simulink model "zbt_transpose"  (Simulink 6.2)
settings: Solver=ode45  StartTime=0.0  StopTime=10.0  RelTol=1e-3
libraries: xbsIndex_r3 x90, fb_library x4
settings Model: LastModifiedBy=mdexter
settings DebuggingCC: SolverPrmCheckMsg=warning

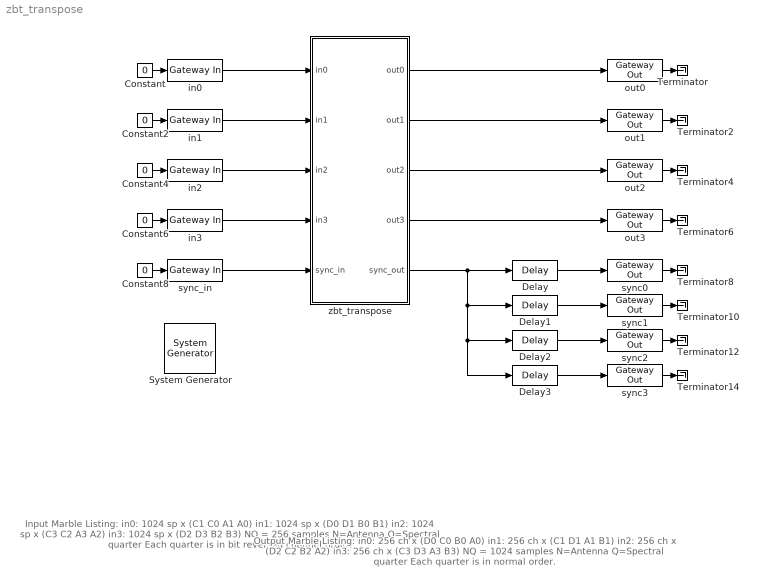
== system zbt_transpose ==
  note: Input Marble Listing:
      |
      | in0: 1024 sp x (C1 C0 A1 A0)
      | in1: 1024 sp x (D0 D1 B0 B1)
      | in2: 1024 sp x (C3 C2 A3 A2)
      | in3: 1024 sp x (D2 D3 B2 B3)
      |
      | NQ = 256 samples
      |
      | N=Antenna
      | Q=Spectral quarter
      |
      | Each quarter is in bit
      | reversed channel order.
  note: Output Marble Listing:
      |
      | in0: 256 ch x (D0 C0 B0 A0)
      | in1: 256 ch x (C1 D1 A1 B1)
      | in2: 256 ch x (D2 C2 B2 A2)
      | in3: 256 ch x (C3 D3 A3 B3)
      |
      | NQ = 1024 samples
      |
      | N=Antenna
      | Q=Spectral quarter
      |
      | Each quarter is in
      | normal order.
  " System Generator" : xbsIndex_r3/ System Generator  Tag=genX  xilinxfamily=Virtex2P  part=xc2vp40  speed=-6  package=ff1152  synthesis_tool=XST  directory=./zbt_transpose_core  testbench=off  simulink_period=1  sysclk_period=100  incr_netlist=off  trim_vbits=Everywhere in SubSystem  dbl_ovrd=According to Block Masks  core_generation=According to Block Masks  run_coregen=off  deprecated_control=off  eval_field=0
      settings: AttributesFormatString=System\nGenerator
  Constant{,2,4,6,8} (5 alike) : Constant  Value=0
  Delay{,1..3} (4 alike) : xbsIndex_r3/Delay  latency=1  reg_retiming=off  explicit_period=off  period=1  en=off  accept_only_valid=off  init_zero=on  dbl_ovrd=off  show_param=off
      settings: xl_area=[0, 0, 0, 0, 0, 0, 0]
  Terminator{,2,4,6,8,10,12,14} (8 alike) : Terminator
  in{0..3} (4 alike) : xbsIndex_r3/Gateway In  arith_type=Unsigned  n_bits=16  bin_pt=0  quantization=Truncate  overflow=Wrap  period=1  timing_constraint=None  locs_specified=off  LOCs={}  needs_fixed_name=off  dbl_ovrd=off  show_param=off
      settings: xl_area=[0, 0, 0, 0, 0, 0, 0]
  out{0..3} (4 alike) : xbsIndex_r3/Gateway Out  output_type=Double  nbits=8  bin_pt=6  arith_type=Boolean  quantization=Truncate  overflow=Wrap  hdl_port=on  timing_constraint=None  locs_specified=off  LOCs={}  needs_fixed_name=off  show_param=off
      settings: xl_area=[0, 0, 0, 0, 0, 0, 0]
  sync{0..3} (4 alike) : xbsIndex_r3/Gateway Out  output_type=Double  nbits=8  bin_pt=6  arith_type=Boolean  quantization=Truncate  overflow=Wrap  hdl_port=on  timing_constraint=None  locs_specified=off  LOCs={}  needs_fixed_name=off  show_param=off
      settings: xl_area=[0, 0, 0, 0, 0, 0, 0]
  sync_in : xbsIndex_r3/Gateway In  arith_type=Boolean  n_bits=16  bin_pt=0  quantization=Truncate  overflow=Wrap  period=1  timing_constraint=None  locs_specified=off  LOCs={}  needs_fixed_name=off  dbl_ovrd=off  show_param=off
      settings: xl_area=[0, 0, 0, 0, 0, 0, 0]
  zbt_transpose : Subsystem
  wires:
  sync_in/1 -> zbt_transpose/5(sync_in)
  zbt_transpose/5(sync_out) -> Delay/1, Delay1/1, Delay3/1, Delay2/1
  Delay/1 -> sync0/1
  Delay1/1 -> sync1/1
  Delay2/1 -> sync2/1
  Delay3/1 -> sync3/1
  Constant/1 -> in0/1
  Constant2/1 -> in1/1
  Constant4/1 -> in2/1
  Constant6/1 -> in3/1
  Constant8/1 -> sync_in/1
  out0/1 -> Terminator/1
  out1/1 -> Terminator2/1
  out2/1 -> Terminator4/1
  out3/1 -> Terminator6/1
  sync0/1 -> Terminator8/1
  sync1/1 -> Terminator10/1
  sync2/1 -> Terminator12/1
  sync3/1 -> Terminator14/1
  in0/1 -> zbt_transpose/1(in0)
  in1/1 -> zbt_transpose/2(in1)
  in2/1 -> zbt_transpose/3(in2)
  in3/1 -> zbt_transpose/4(in3)
  zbt_transpose/1(out0) -> out0/1
  zbt_transpose/2(out1) -> out1/1
  zbt_transpose/3(out2) -> out2/1
  zbt_transpose/4(out3) -> out3/1

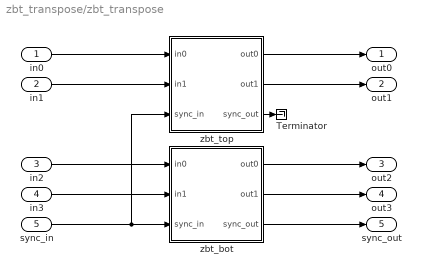
== system zbt_transpose/zbt_transpose ==
  in0 : Inport  Port=1  LatchInput=off
  in1 : Inport  Port=2  LatchInput=off
  in2 : Inport  Port=3  LatchInput=off
  in3 : Inport  Port=4  LatchInput=off
  sync_in : Inport  Port=5  LatchInput=off
  Terminator : Terminator
  zbt_bot : Subsystem
  zbt_top : Subsystem
  out0 : Outport
  out1 : Outport  Port=2
  out2 : Outport  Port=3
  out3 : Outport  Port=4
  sync_out : Outport  Port=5
  wires:
  zbt_top/1(out0) -> out0/1
  in0/1 -> zbt_top/1(in0)
  in1/1 -> zbt_top/2(in1)
  zbt_top/2(out1) -> out1/1
  zbt_bot/1(out0) -> out2/1
  in2/1 -> zbt_bot/1(in0)
  in3/1 -> zbt_bot/2(in1)
  zbt_bot/2(out1) -> out3/1
  sync_in/1 -> zbt_bot/3(sync_in), zbt_top/3(sync_in)
  zbt_bot/3(sync_out) -> sync_out/1
  zbt_top/3(sync_out) -> Terminator/1

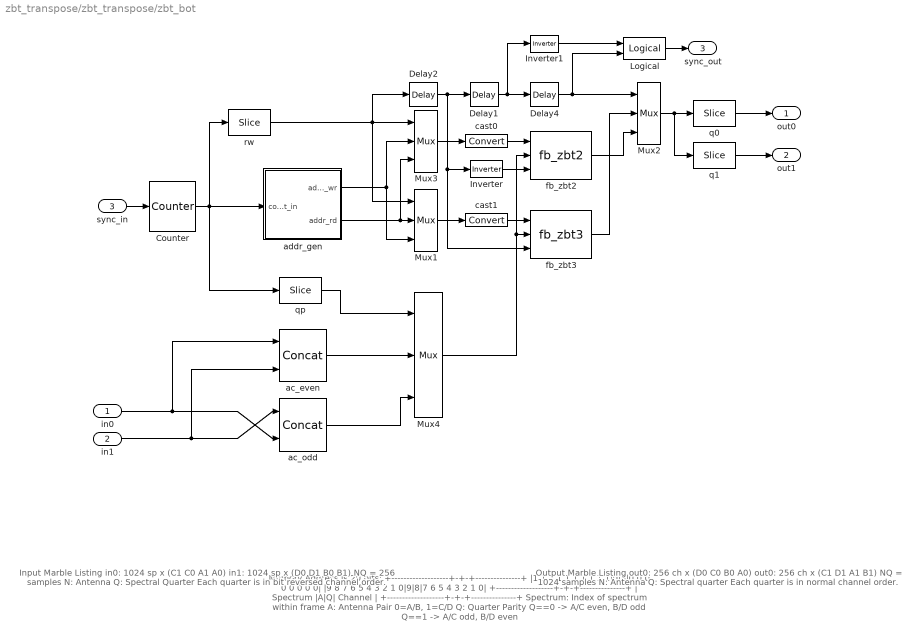
== system zbt_transpose/zbt_transpose/zbt_bot ==
  note: Memory Address is 20 bits:
      | +-------------------+-+-+---------------+
      | |1 1 1 1 1 1 1 1 1 1|0|0|0 0 0 0 0 0 0 0|
      | |9 8 7 6 5 4 3 2 1 0|9|8|7 6 5 4 3 2 1 0|
      | +-------------------+-+-+---------------+
      | |     Spectrum      |A|Q|    Channel    |
      | +-------------------+-+-+---------------+
      |
      | Spectrum: Index of spectrum within frame
      | A: Antenna Pair 0=A/B, 1=C/D
      | Q: Quarter Parity
      | Q==0 -> A/C even, B/D odd
      | Q==1 -> A/C odd, B/D even
  note: Input Marble Listing
      | in0: 1024 sp x (C1 C0 A1 A0)
      | in1: 1024 sp x (D0 D1 B0 B1)
      |
      | NQ = 256 samples
      |
      | N: Antenna
      | Q: Spectral Quarter
      |
      | Each quarter is in bit
      | reversed channel order.
  note: Output Marble Listing
      | out0: 256 ch x (D0 C0 B0 A0)
      | out0: 256 ch x (C1 D1 A1 B1)
      |
      | NQ = 1024 samples
      |
      | N: Antenna
      | Q: Spectral quarter
      |
      | Each quarter is in
      | normal channel order.
  in0 : Inport  Port=1  LatchInput=off
  in1 : Inport  Port=2  LatchInput=off
  sync_in : Inport  Port=3  LatchInput=off
  Counter : xbsIndex_r3/Counter  cnt_type=Free Running  n_bits=21  bin_pt=0  arith_type=Unsigned  start_count=0  cnt_to=Inf  cnt_by_val=1  operation=Up  explicit_period=on  period=1  load_pin=off  rst=on  en=off  dbl_ovrd=off  show_param=off  use_rpm=on  gen_core=off
      settings: xl_area=[0, 0, 0, 0, 0, 0, 0]
  Delay1 : xbsIndex_r3/Delay  latency=3  reg_retiming=off  explicit_period=off  period=1  en=off  accept_only_valid=off  init_zero=on  dbl_ovrd=off  show_param=off
      settings: xl_area=[0, 0, 0, 0, 0, 0, 0]
  Delay2 : xbsIndex_r3/Delay  latency=1  reg_retiming=off  explicit_period=off  period=1  en=off  accept_only_valid=off  init_zero=on  dbl_ovrd=off  show_param=off
      settings: xl_area=[0, 0, 0, 0, 0, 0, 0]
  Delay4 : xbsIndex_r3/Delay  latency=1  reg_retiming=off  explicit_period=off  period=1  en=off  accept_only_valid=off  init_zero=on  dbl_ovrd=off  show_param=off
      settings: xl_area=[0, 0, 0, 0, 0, 0, 0]
  Inverter : xbsIndex_r3/Inverter  latency=0  explicit_period=off  period=1  en=off  dbl_ovrd=off  show_param=off
      settings: xl_area=[0, 0, 0, 0, 0, 0, 0]
  Inverter1 : xbsIndex_r3/Inverter  latency=0  explicit_period=off  period=1  en=off  dbl_ovrd=off  show_param=off
      settings: xl_area=[0, 0, 0, 0, 0, 0, 0]
  Logical : xbsIndex_r3/Logical  logical_function=AND  inputs=2  precision=Full  arith_type=Unsigned  n_bits=8  bin_pt=2  align_bp=on  latency=1  explicit_period=off  period=1  en=off  dbl_ovrd=off  show_param=off
      settings: xl_area=[0, 0, 0, 0, 0, 0, 0]
  Mux1 : xbsIndex_r3/Mux  inputs=2  precision=Full  arith_type="Signed  (2's comp)"  n_bits=8  bin_pt=2  quantization=Truncate  overflow=Wrap  latency=1  explicit_period=off  period=1  en=off  dbl_ovrd=off  show_param=on  mux_type=off  use_rpm=off  gen_core=off
      settings: xl_area=[0, 0, 0, 0, 0, 0, 0]
  Mux2 : xbsIndex_r3/Mux  inputs=2  precision=Full  arith_type="Signed  (2's comp)"  n_bits=8  bin_pt=2  quantization=Truncate  overflow=Wrap  latency=1  explicit_period=off  period=1  en=off  dbl_ovrd=off  show_param=off  mux_type=off  use_rpm=off  gen_core=off
      settings: xl_area=[0, 0, 0, 0, 0, 0, 0]
  Mux3 : xbsIndex_r3/Mux  inputs=2  precision=Full  arith_type="Signed  (2's comp)"  n_bits=8  bin_pt=2  quantization=Truncate  overflow=Wrap  latency=1  explicit_period=off  period=1  en=off  dbl_ovrd=off  show_param=on  mux_type=off  use_rpm=off  gen_core=off
      settings: xl_area=[0, 0, 0, 0, 0, 0, 0]
  Mux4 : xbsIndex_r3/Mux  inputs=2  precision=Full  arith_type="Signed  (2's comp)"  n_bits=8  bin_pt=2  quantization=Truncate  overflow=Wrap  latency=1  explicit_period=off  period=1  en=off  dbl_ovrd=off  show_param=on  mux_type=off  use_rpm=off  gen_core=off
      settings: xl_area=[0, 0, 0, 0, 0, 0, 0]
  ac_even : xbsIndex_r3/Concat  num_inputs=2  explicit_period=off  period=1  dbl_ovrd=off
  ac_odd : xbsIndex_r3/Concat  num_inputs=2  explicit_period=off  period=1  dbl_ovrd=off
  addr_gen : Subsystem
  cast0 : xbsIndex_r3/Convert  arith_type=Unsigned  n_bits=23  bin_pt=0  quantization=Truncate  overflow=Wrap  latency=0  explicit_period=off  period=1  dbl_ovrd=off  show_param=off  inserted_by_tool=off  pipeline=off
      settings: xl_area=[0, 0, 0, 0, 0, 0, 0]
  cast1 : xbsIndex_r3/Convert  arith_type=Unsigned  n_bits=23  bin_pt=0  quantization=Truncate  overflow=Wrap  latency=0  explicit_period=off  period=1  dbl_ovrd=off  show_param=off  inserted_by_tool=off  pipeline=off
      settings: xl_area=[0, 0, 0, 0, 0, 0, 0]
  fb_zbt2 : fb_library/fb_zbt2
      link override fb_zbt2_8m: BlockChoice=zbt_8m_sim
  fb_zbt3 : fb_library/fb_zbt3
      link override fb_zbt3_8m: BlockChoice=zbt_8m_sim
  q0 : xbsIndex_r3/Slice  mode=Upper Bit Location + Width  nbits=16  bit1=0  base1=MSB of Input  bit0=0  base0=LSB of Input  boolean_output=off  explicit_period=off  period=1  dbl_ovrd=off
  q1 : xbsIndex_r3/Slice  mode=Lower Bit Location + Width  nbits=16  bit1=0  base1=MSB of Input  bit0=0  base0=LSB of Input  boolean_output=off  explicit_period=off  period=1  dbl_ovrd=off
  qp : xbsIndex_r3/Slice  mode=Lower Bit Location + Width  nbits=1  bit1=0  base1=MSB of Input  bit0=8  base0=LSB of Input  boolean_output=off  explicit_period=off  period=1  dbl_ovrd=off
  rw : xbsIndex_r3/Slice  mode=Upper Bit Location + Width  nbits=1  bit1=0  base1=MSB of Input  bit0=0  base0=LSB of Input  boolean_output=on  explicit_period=off  period=1  dbl_ovrd=off
  out0 : Outport
  out1 : Outport  Port=2
  sync_out : Outport  Port=3
  wires:
  Inverter/1 -> fb_zbt2/3
  Delay1/1 -> Delay4/1, Inverter1/1
  fb_zbt2/1 -> Mux2/3
  fb_zbt3/1 -> Mux2/2
  Mux1/1 -> cast1/1
  Mux3/1 -> cast0/1
  addr_gen/2(addr_rd) -> Mux1/2, Mux3/3
  addr_gen/1(addr_wr) -> Mux1/3, Mux3/2
  rw/1 -> Mux1/1, Mux3/1, Delay2/1
  Counter/1 -> rw/1, addr_gen/1(count_in), qp/1
  Inverter1/1 -> Logical/1
  Delay4/1 -> Logical/2, Mux2/1
  cast0/1 -> fb_zbt2/1
  cast1/1 -> fb_zbt3/1
  Logical/1 -> sync_out/1
  Mux2/1 -> q0/1, q1/1
  sync_in/1 -> Counter/1
  Delay2/1 -> Inverter/1, fb_zbt3/3, Delay1/1
  Mux4/1 -> fb_zbt2/2, fb_zbt3/2
  in1/1 -> ac_odd/1, ac_even/2
  in0/1 -> ac_odd/2, ac_even/1
  ac_even/1 -> Mux4/2
  ac_odd/1 -> Mux4/3
  qp/1 -> Mux4/1
  q0/1 -> out0/1
  q1/1 -> out1/1

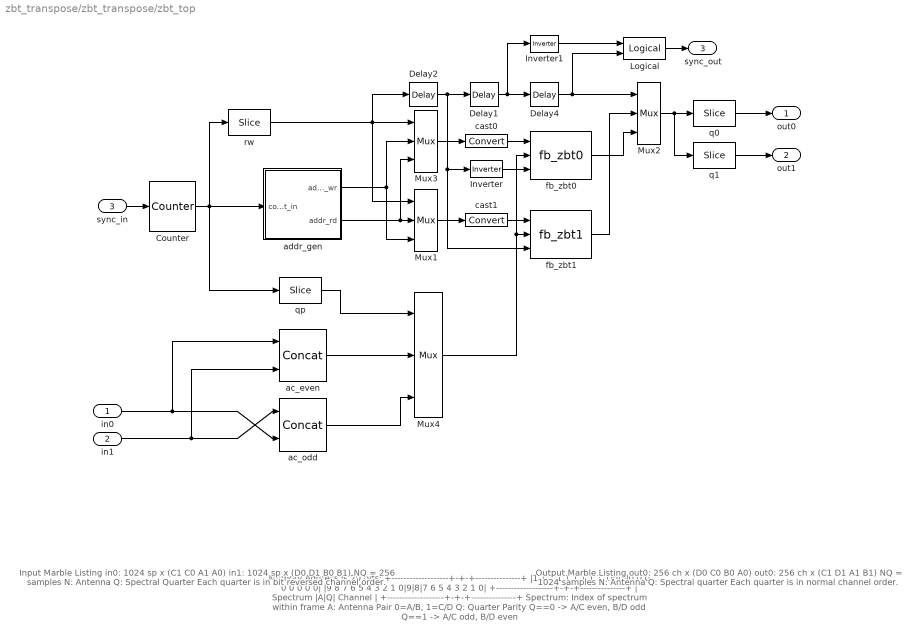
== system zbt_transpose/zbt_transpose/zbt_top ==
  note: Memory Address is 20 bits:
      | +-------------------+-+-+---------------+
      | |1 1 1 1 1 1 1 1 1 1|0|0|0 0 0 0 0 0 0 0|
      | |9 8 7 6 5 4 3 2 1 0|9|8|7 6 5 4 3 2 1 0|
      | +-------------------+-+-+---------------+
      | |     Spectrum      |A|Q|    Channel    |
      | +-------------------+-+-+---------------+
      |
      | Spectrum: Index of spectrum within frame
      | A: Antenna Pair 0=A/B, 1=C/D
      | Q: Quarter Parity
      | Q==0 -> A/C even, B/D odd
      | Q==1 -> A/C odd, B/D even
  note: Input Marble Listing
      | in0: 1024 sp x (C1 C0 A1 A0)
      | in1: 1024 sp x (D0 D1 B0 B1)
      |
      | NQ = 256 samples
      |
      | N: Antenna
      | Q: Spectral Quarter
      |
      | Each quarter is in bit
      | reversed channel order.
  note: Output Marble Listing
      | out0: 256 ch x (D0 C0 B0 A0)
      | out0: 256 ch x (C1 D1 A1 B1)
      |
      | NQ = 1024 samples
      |
      | N: Antenna
      | Q: Spectral quarter
      |
      | Each quarter is in
      | normal channel order.
  in0 : Inport  Port=1  LatchInput=off
  in1 : Inport  Port=2  LatchInput=off
  sync_in : Inport  Port=3  LatchInput=off
  Counter : xbsIndex_r3/Counter  cnt_type=Free Running  n_bits=21  bin_pt=0  arith_type=Unsigned  start_count=0  cnt_to=Inf  cnt_by_val=1  operation=Up  explicit_period=on  period=1  load_pin=off  rst=on  en=off  dbl_ovrd=off  show_param=off  use_rpm=on  gen_core=off
      settings: xl_area=[0, 0, 0, 0, 0, 0, 0]
  Delay1 : xbsIndex_r3/Delay  latency=3  reg_retiming=off  explicit_period=off  period=1  en=off  accept_only_valid=off  init_zero=on  dbl_ovrd=off  show_param=off
      settings: xl_area=[0, 0, 0, 0, 0, 0, 0]
  Delay2 : xbsIndex_r3/Delay  latency=1  reg_retiming=off  explicit_period=off  period=1  en=off  accept_only_valid=off  init_zero=on  dbl_ovrd=off  show_param=off
      settings: xl_area=[0, 0, 0, 0, 0, 0, 0]
  Delay4 : xbsIndex_r3/Delay  latency=1  reg_retiming=off  explicit_period=off  period=1  en=off  accept_only_valid=off  init_zero=on  dbl_ovrd=off  show_param=off
      settings: xl_area=[0, 0, 0, 0, 0, 0, 0]
  Inverter : xbsIndex_r3/Inverter  latency=0  explicit_period=off  period=1  en=off  dbl_ovrd=off  show_param=off
      settings: xl_area=[0, 0, 0, 0, 0, 0, 0]
  Inverter1 : xbsIndex_r3/Inverter  latency=0  explicit_period=off  period=1  en=off  dbl_ovrd=off  show_param=off
      settings: xl_area=[0, 0, 0, 0, 0, 0, 0]
  Logical : xbsIndex_r3/Logical  logical_function=AND  inputs=2  precision=Full  arith_type=Unsigned  n_bits=8  bin_pt=2  align_bp=on  latency=1  explicit_period=off  period=1  en=off  dbl_ovrd=off  show_param=off
      settings: xl_area=[0, 0, 0, 0, 0, 0, 0]
  Mux1 : xbsIndex_r3/Mux  inputs=2  precision=Full  arith_type="Signed  (2's comp)"  n_bits=8  bin_pt=2  quantization=Truncate  overflow=Wrap  latency=1  explicit_period=off  period=1  en=off  dbl_ovrd=off  show_param=on  mux_type=off  use_rpm=off  gen_core=off
      settings: xl_area=[0, 0, 0, 0, 0, 0, 0]
  Mux2 : xbsIndex_r3/Mux  inputs=2  precision=Full  arith_type="Signed  (2's comp)"  n_bits=8  bin_pt=2  quantization=Truncate  overflow=Wrap  latency=1  explicit_period=off  period=1  en=off  dbl_ovrd=off  show_param=off  mux_type=off  use_rpm=off  gen_core=off
      settings: xl_area=[0, 0, 0, 0, 0, 0, 0]
  Mux3 : xbsIndex_r3/Mux  inputs=2  precision=Full  arith_type="Signed  (2's comp)"  n_bits=8  bin_pt=2  quantization=Truncate  overflow=Wrap  latency=1  explicit_period=off  period=1  en=off  dbl_ovrd=off  show_param=on  mux_type=off  use_rpm=off  gen_core=off
      settings: xl_area=[0, 0, 0, 0, 0, 0, 0]
  Mux4 : xbsIndex_r3/Mux  inputs=2  precision=Full  arith_type="Signed  (2's comp)"  n_bits=8  bin_pt=2  quantization=Truncate  overflow=Wrap  latency=1  explicit_period=off  period=1  en=off  dbl_ovrd=off  show_param=on  mux_type=off  use_rpm=off  gen_core=off
      settings: xl_area=[0, 0, 0, 0, 0, 0, 0]
  ac_even : xbsIndex_r3/Concat  num_inputs=2  explicit_period=off  period=1  dbl_ovrd=off
  ac_odd : xbsIndex_r3/Concat  num_inputs=2  explicit_period=off  period=1  dbl_ovrd=off
  addr_gen : Subsystem
  cast0 : xbsIndex_r3/Convert  arith_type=Unsigned  n_bits=23  bin_pt=0  quantization=Truncate  overflow=Wrap  latency=0  explicit_period=off  period=1  dbl_ovrd=off  show_param=off  inserted_by_tool=off  pipeline=off
      settings: xl_area=[0, 0, 0, 0, 0, 0, 0]
  cast1 : xbsIndex_r3/Convert  arith_type=Unsigned  n_bits=23  bin_pt=0  quantization=Truncate  overflow=Wrap  latency=0  explicit_period=off  period=1  dbl_ovrd=off  show_param=off  inserted_by_tool=off  pipeline=off
      settings: xl_area=[0, 0, 0, 0, 0, 0, 0]
  fb_zbt0 : fb_library/fb_zbt0
      link override fb_zbt0_8m: BlockChoice=zbt_8m_sim
  fb_zbt1 : fb_library/fb_zbt1
      link override fb_zbt1_8m: BlockChoice=zbt_8m_sim
  q0 : xbsIndex_r3/Slice  mode=Upper Bit Location + Width  nbits=16  bit1=0  base1=MSB of Input  bit0=0  base0=LSB of Input  boolean_output=off  explicit_period=off  period=1  dbl_ovrd=off
  q1 : xbsIndex_r3/Slice  mode=Lower Bit Location + Width  nbits=16  bit1=0  base1=MSB of Input  bit0=0  base0=LSB of Input  boolean_output=off  explicit_period=off  period=1  dbl_ovrd=off
  qp : xbsIndex_r3/Slice  mode=Lower Bit Location + Width  nbits=1  bit1=0  base1=MSB of Input  bit0=8  base0=LSB of Input  boolean_output=off  explicit_period=off  period=1  dbl_ovrd=off
  rw : xbsIndex_r3/Slice  mode=Upper Bit Location + Width  nbits=1  bit1=0  base1=MSB of Input  bit0=0  base0=LSB of Input  boolean_output=on  explicit_period=off  period=1  dbl_ovrd=off
  out0 : Outport
  out1 : Outport  Port=2
  sync_out : Outport  Port=3
  wires:
  Inverter/1 -> fb_zbt0/3
  Delay1/1 -> Delay4/1, Inverter1/1
  fb_zbt0/1 -> Mux2/3
  fb_zbt1/1 -> Mux2/2
  Mux1/1 -> cast1/1
  Mux3/1 -> cast0/1
  addr_gen/2(addr_rd) -> Mux1/2, Mux3/3
  addr_gen/1(addr_wr) -> Mux1/3, Mux3/2
  rw/1 -> Mux1/1, Mux3/1, Delay2/1
  Counter/1 -> rw/1, addr_gen/1(count_in), qp/1
  Inverter1/1 -> Logical/1
  Delay4/1 -> Logical/2, Mux2/1
  cast0/1 -> fb_zbt0/1
  cast1/1 -> fb_zbt1/1
  Logical/1 -> sync_out/1
  Mux2/1 -> q0/1, q1/1
  sync_in/1 -> Counter/1
  Delay2/1 -> Inverter/1, fb_zbt1/3, Delay1/1
  Mux4/1 -> fb_zbt1/2, fb_zbt0/2
  in1/1 -> ac_odd/1, ac_even/2
  in0/1 -> ac_odd/2, ac_even/1
  ac_even/1 -> Mux4/2
  ac_odd/1 -> Mux4/3
  qp/1 -> Mux4/1
  q0/1 -> out0/1
  q1/1 -> out1/1

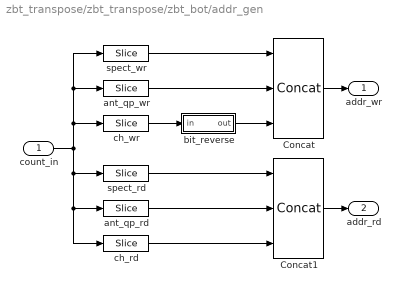
== system zbt_transpose/zbt_transpose/zbt_bot/addr_gen ==
  count_in : Inport  Port=1  LatchInput=off
  Concat : xbsIndex_r3/Concat  num_inputs=3  explicit_period=off  period=1  dbl_ovrd=off
  Concat1 : xbsIndex_r3/Concat  num_inputs=3  explicit_period=off  period=1  dbl_ovrd=off
  ant_qp_rd : xbsIndex_r3/Slice  mode=Lower Bit Location + Width  nbits=2  bit1=10  base1=MSB of Input  bit0=10  base0=LSB of Input  boolean_output=off  explicit_period=off  period=1  dbl_ovrd=off
  ant_qp_wr : xbsIndex_r3/Slice  mode=Lower Bit Location + Width  nbits=2  bit1=10  base1=MSB of Input  bit0=8  base0=LSB of Input  boolean_output=off  explicit_period=off  period=1  dbl_ovrd=off
  bit_reverse : Subsystem  mask(Bit Reversal){n_bits=8}
      mask prompts: n_bits "Number of Bits"
      mask help: Reverses the bit order of the input. Input must be unsigned with binary point at position 0. Costs nothing in hardware.
      mask init:
      | bit_reverse_init(gcb,n_bits);
      settings: AttributesFormatString=8 bits
      mask Help:
      | <pre>
      | Description::
      | 
      | Reverses the bit order of the input.
      | 
      | Input must be unsigned with binary point at position 0.
      | 
      | Costs nothing in hardware.
      | 
      | Mask Parameters::
      | 
      | Number of Bits (n_bits): Specifies the width of the input.
      | </pre>
  ch_rd : xbsIndex_r3/Slice  mode=Lower Bit Location + Width  nbits=8  bit1=10  base1=MSB of Input  bit0=12  base0=LSB of Input  boolean_output=off  explicit_period=off  period=1  dbl_ovrd=off
  ch_wr : xbsIndex_r3/Slice  mode=Lower Bit Location + Width  nbits=8  bit1=10  base1=MSB of Input  bit0=0  base0=LSB of Input  boolean_output=off  explicit_period=off  period=1  dbl_ovrd=off
  spect_rd : xbsIndex_r3/Slice  mode=Lower Bit Location + Width  nbits=10  bit1=10  base1=MSB of Input  bit0=0  base0=LSB of Input  boolean_output=off  explicit_period=off  period=1  dbl_ovrd=off
  spect_wr : xbsIndex_r3/Slice  mode=Lower Bit Location + Width  nbits=10  bit1=10  base1=MSB of Input  bit0=10  base0=LSB of Input  boolean_output=off  explicit_period=off  period=1  dbl_ovrd=off
  addr_wr : Outport
  addr_rd : Outport  Port=2
  wires:
  spect_wr/1 -> Concat/1
  Concat/1 -> addr_wr/1
  Concat1/1 -> addr_rd/1
  ant_qp_wr/1 -> Concat/2
  ch_wr/1 -> bit_reverse/1(in)
  spect_rd/1 -> Concat1/1
  ant_qp_rd/1 -> Concat1/2
  ch_rd/1 -> Concat1/3
  count_in/1 -> ch_wr/1, spect_wr/1, ant_qp_wr/1, ch_rd/1, ant_qp_rd/1, spect_rd/1
  bit_reverse/1(out) -> Concat/3

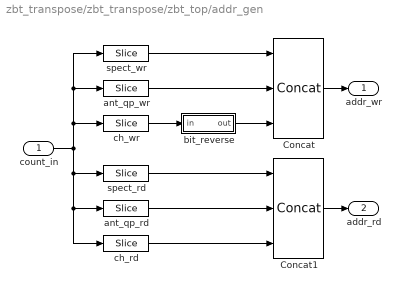
== system zbt_transpose/zbt_transpose/zbt_top/addr_gen ==
  count_in : Inport  Port=1  LatchInput=off
  Concat : xbsIndex_r3/Concat  num_inputs=3  explicit_period=off  period=1  dbl_ovrd=off
  Concat1 : xbsIndex_r3/Concat  num_inputs=3  explicit_period=off  period=1  dbl_ovrd=off
  ant_qp_rd : xbsIndex_r3/Slice  mode=Lower Bit Location + Width  nbits=2  bit1=10  base1=MSB of Input  bit0=10  base0=LSB of Input  boolean_output=off  explicit_period=off  period=1  dbl_ovrd=off
  ant_qp_wr : xbsIndex_r3/Slice  mode=Lower Bit Location + Width  nbits=2  bit1=10  base1=MSB of Input  bit0=8  base0=LSB of Input  boolean_output=off  explicit_period=off  period=1  dbl_ovrd=off
  bit_reverse : Subsystem  mask(Bit Reversal){n_bits=8}
      mask prompts: n_bits "Number of Bits"
      mask help: Reverses the bit order of the input. Input must be unsigned with binary point at position 0. Costs nothing in hardware.
      mask init:
      | bit_reverse_init(gcb,n_bits);
      settings: AttributesFormatString=8 bits
      mask Help:
      | <pre>
      | Description::
      | 
      | Reverses the bit order of the input.
      | 
      | Input must be unsigned with binary point at position 0.
      | 
      | Costs nothing in hardware.
      | 
      | Mask Parameters::
      | 
      | Number of Bits (n_bits): Specifies the width of the input.
      | </pre>
  ch_rd : xbsIndex_r3/Slice  mode=Lower Bit Location + Width  nbits=8  bit1=10  base1=MSB of Input  bit0=12  base0=LSB of Input  boolean_output=off  explicit_period=off  period=1  dbl_ovrd=off
  ch_wr : xbsIndex_r3/Slice  mode=Lower Bit Location + Width  nbits=8  bit1=10  base1=MSB of Input  bit0=0  base0=LSB of Input  boolean_output=off  explicit_period=off  period=1  dbl_ovrd=off
  spect_rd : xbsIndex_r3/Slice  mode=Lower Bit Location + Width  nbits=10  bit1=10  base1=MSB of Input  bit0=0  base0=LSB of Input  boolean_output=off  explicit_period=off  period=1  dbl_ovrd=off
  spect_wr : xbsIndex_r3/Slice  mode=Lower Bit Location + Width  nbits=10  bit1=10  base1=MSB of Input  bit0=10  base0=LSB of Input  boolean_output=off  explicit_period=off  period=1  dbl_ovrd=off
  addr_wr : Outport
  addr_rd : Outport  Port=2
  wires:
  spect_wr/1 -> Concat/1
  Concat/1 -> addr_wr/1
  Concat1/1 -> addr_rd/1
  ant_qp_wr/1 -> Concat/2
  ch_wr/1 -> bit_reverse/1(in)
  spect_rd/1 -> Concat1/1
  ant_qp_rd/1 -> Concat1/2
  ch_rd/1 -> Concat1/3
  count_in/1 -> ch_wr/1, spect_wr/1, ant_qp_wr/1, ch_rd/1, ant_qp_rd/1, spect_rd/1
  bit_reverse/1(out) -> Concat/3

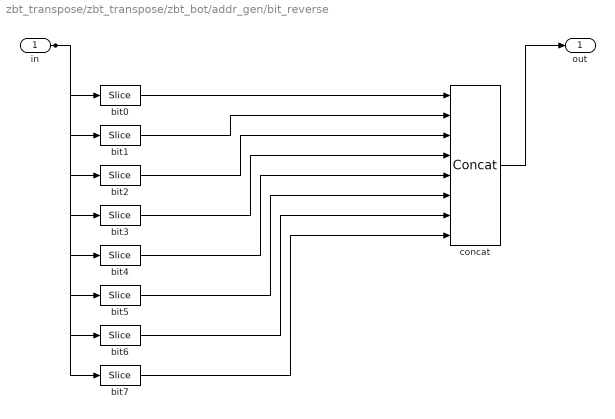
== system zbt_transpose/zbt_transpose/zbt_bot/addr_gen/bit_reverse ==
  in : Inport  Port=1  LatchInput=off
  bit0 : xbsIndex_r3/Slice  mode=Lower Bit Location + Width  nbits=1  bit1=0  base1=MSB of Input  bit0=0  base0=LSB of Input  boolean_output=off  explicit_period=off  period=1  dbl_ovrd=off
  bit1 : xbsIndex_r3/Slice  mode=Lower Bit Location + Width  nbits=1  bit1=0  base1=MSB of Input  bit0=1  base0=LSB of Input  boolean_output=off  explicit_period=off  period=1  dbl_ovrd=off
  bit2 : xbsIndex_r3/Slice  mode=Lower Bit Location + Width  nbits=1  bit1=0  base1=MSB of Input  bit0=2  base0=LSB of Input  boolean_output=off  explicit_period=off  period=1  dbl_ovrd=off
  bit3 : xbsIndex_r3/Slice  mode=Lower Bit Location + Width  nbits=1  bit1=0  base1=MSB of Input  bit0=3  base0=LSB of Input  boolean_output=off  explicit_period=off  period=1  dbl_ovrd=off
  bit4 : xbsIndex_r3/Slice  mode=Lower Bit Location + Width  nbits=1  bit1=0  base1=MSB of Input  bit0=4  base0=LSB of Input  boolean_output=off  explicit_period=off  period=1  dbl_ovrd=off
  bit5 : xbsIndex_r3/Slice  mode=Lower Bit Location + Width  nbits=1  bit1=0  base1=MSB of Input  bit0=5  base0=LSB of Input  boolean_output=off  explicit_period=off  period=1  dbl_ovrd=off
  bit6 : xbsIndex_r3/Slice  mode=Lower Bit Location + Width  nbits=1  bit1=0  base1=MSB of Input  bit0=6  base0=LSB of Input  boolean_output=off  explicit_period=off  period=1  dbl_ovrd=off
  bit7 : xbsIndex_r3/Slice  mode=Lower Bit Location + Width  nbits=1  bit1=0  base1=MSB of Input  bit0=7  base0=LSB of Input  boolean_output=off  explicit_period=off  period=1  dbl_ovrd=off
  concat : xbsIndex_r3/Concat  num_inputs=8  explicit_period=off  period=1  dbl_ovrd=off
  out : Outport
  wires:
  in/1 -> bit7/1, bit6/1, bit5/1, bit4/1, bit3/1, bit2/1, bit1/1, bit0/1
  bit7/1 -> concat/8
  bit6/1 -> concat/7
  bit5/1 -> concat/6
  bit4/1 -> concat/5
  bit3/1 -> concat/4
  bit2/1 -> concat/3
  bit1/1 -> concat/2
  bit0/1 -> concat/1
  concat/1 -> out/1

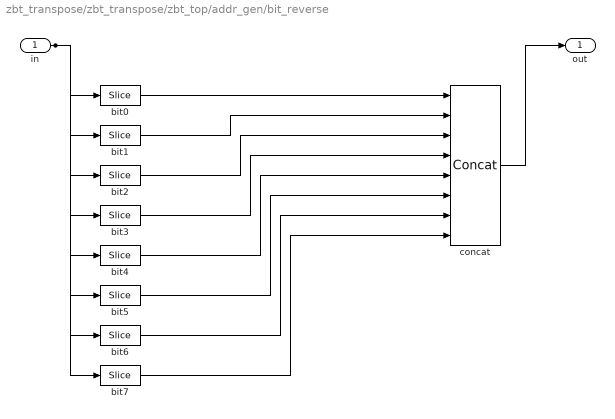
== system zbt_transpose/zbt_transpose/zbt_top/addr_gen/bit_reverse ==
  in : Inport  Port=1  LatchInput=off
  bit0 : xbsIndex_r3/Slice  mode=Lower Bit Location + Width  nbits=1  bit1=0  base1=MSB of Input  bit0=0  base0=LSB of Input  boolean_output=off  explicit_period=off  period=1  dbl_ovrd=off
  bit1 : xbsIndex_r3/Slice  mode=Lower Bit Location + Width  nbits=1  bit1=0  base1=MSB of Input  bit0=1  base0=LSB of Input  boolean_output=off  explicit_period=off  period=1  dbl_ovrd=off
  bit2 : xbsIndex_r3/Slice  mode=Lower Bit Location + Width  nbits=1  bit1=0  base1=MSB of Input  bit0=2  base0=LSB of Input  boolean_output=off  explicit_period=off  period=1  dbl_ovrd=off
  bit3 : xbsIndex_r3/Slice  mode=Lower Bit Location + Width  nbits=1  bit1=0  base1=MSB of Input  bit0=3  base0=LSB of Input  boolean_output=off  explicit_period=off  period=1  dbl_ovrd=off
  bit4 : xbsIndex_r3/Slice  mode=Lower Bit Location + Width  nbits=1  bit1=0  base1=MSB of Input  bit0=4  base0=LSB of Input  boolean_output=off  explicit_period=off  period=1  dbl_ovrd=off
  bit5 : xbsIndex_r3/Slice  mode=Lower Bit Location + Width  nbits=1  bit1=0  base1=MSB of Input  bit0=5  base0=LSB of Input  boolean_output=off  explicit_period=off  period=1  dbl_ovrd=off
  bit6 : xbsIndex_r3/Slice  mode=Lower Bit Location + Width  nbits=1  bit1=0  base1=MSB of Input  bit0=6  base0=LSB of Input  boolean_output=off  explicit_period=off  period=1  dbl_ovrd=off
  bit7 : xbsIndex_r3/Slice  mode=Lower Bit Location + Width  nbits=1  bit1=0  base1=MSB of Input  bit0=7  base0=LSB of Input  boolean_output=off  explicit_period=off  period=1  dbl_ovrd=off
  concat : xbsIndex_r3/Concat  num_inputs=8  explicit_period=off  period=1  dbl_ovrd=off
  out : Outport
  wires:
  in/1 -> bit7/1, bit6/1, bit5/1, bit4/1, bit3/1, bit2/1, bit1/1, bit0/1
  bit7/1 -> concat/8
  bit6/1 -> concat/7
  bit5/1 -> concat/6
  bit4/1 -> concat/5
  bit3/1 -> concat/4
  bit2/1 -> concat/3
  bit1/1 -> concat/2
  bit0/1 -> concat/1
  concat/1 -> out/1
